simulink model "gates"  (R2024a)
settings: Solver=VariableStepAuto  StartTime=0.0  StopTime=10.0  RelTol=1e-3
libraries: simulink x6
settings Model: Creator=lokes  LastModifiedBy=tusha
settings RTWCC: GPUComputeCapability=3.5

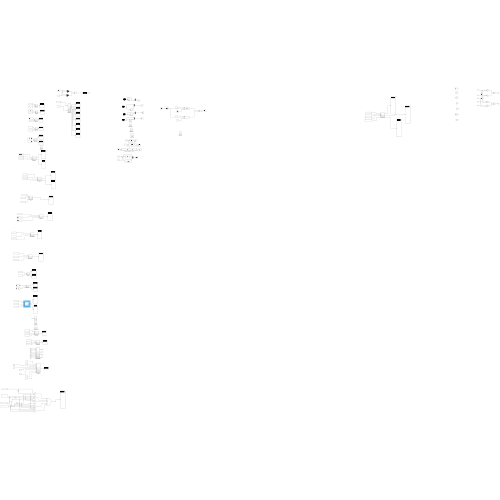
[thumbnail: Simulink's stored preview of the top-level diagram]
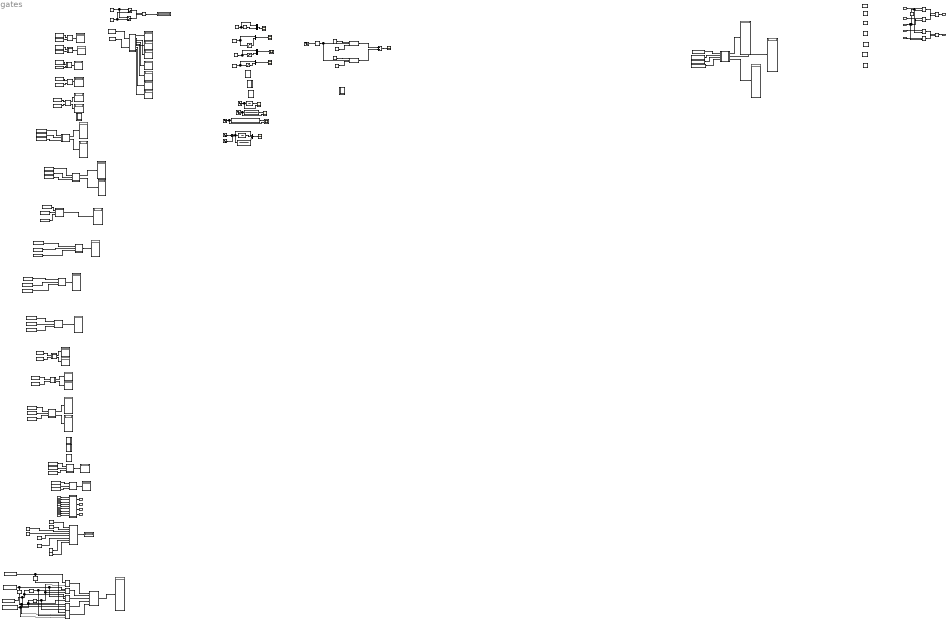
== system gates ==
  note: [numd, dend]=bilinear([1],[1 1.414 1],1)
  In1 : Inport
  In2 : Inport  Port=2
  In3 : Inport  Port=3
  In4 : Inport  Port=4
  In5 : Inport  Port=5
  In6 : Inport  Port=6
  In7 : Inport  Port=7
  In8 : Inport  Port=8
  In10 : Inport  Port=9
  In9 : Inport  Port=10
  In11 : Inport  Port=11
  In12 : Inport  Port=12
  In13 : Inport  Port=13
  In14 : Inport  Port=14
  2:1MUX(Basic) : Subsystem
  2:1MUX(NAND) : Subsystem
  3NOR USING 2NOR : Subsystem
  4:1MUX : Subsystem
  4BIT(2:1)MUXNAND : Subsystem
  A+B+C : Subsystem
  ABC : Subsystem
  AC+B : Subsystem
  Absorption : Subsystem
  Add : Sum
  BASIC GATES : Subsystem
  Bus Creator{,1..3} (4 alike) : BusCreator  Inputs=2
  Bus Creator4 : BusCreator  Inputs=3
  Constant{,40..41,55} (4 alike) : Constant  Value=0
  Constant{1,39,49..54,56} (9 alike) : Constant
  Constant{2,4,6,8,10,12,32,34,45,48} (10 alike) : Constant  Value=[0 0 1 1]
  Constant{3,5,7,9,11,13,33,35} (8 alike) : Constant  Value=[0 1 0 1]
  Constant{14,17,20,23,26,29,36} (7 alike) : Constant  Value=[0 0 0 0 1 1 1 1]
  Constant{15,18,21,24,27,30,37} (7 alike) : Constant  Value=[0 0 1 1 0 0 1 1]
  Constant{16,19,22,25,28,31,38} (7 alike) : Constant  Value=[0 1 0 1 0 1 0 1]
  Constant42 : Constant  Value=-1
  Constant43 : Constant  Value=[0 1 0 0]
  Constant44 : Constant  Value=[0 0 0 1]
  Constant46 : Constant  Value=[0 1 0 0]
  Constant47 : Constant  Value=[0 0 0 1]
  Constant57 : Constant  Value=[0 0 0 0 0 0 0 0 1 1 1 1 1 1 1 1]
  Constant58 : Constant  Value=[0 0 0 0 1 1 1 1 0 0 0 0 1 1 1 1]
  Constant59 : Constant  Value=[0 0 1 1 0 0 1 1 0 0 1 1 0 0 1 1]
  Constant60 : Constant  Value=[0 1 0 1 0 1 0 1 0 1 0 1 0 1 0 1]
  Constant61 : Constant  Value=[0 0 0 0 0 0 0 0 1 1 1 1 1 1 1 1]
  Constant62 : Constant  Value=[0 0 0 0 1 1 1 1 0 0 0 0 1 1 1 1]
  Constant63 : Constant  Value=[0 0 1 1 0 0 1 1 0 0 1 1 0 0 1 1]
  Constant64 : Constant  Value=[0 1 0 1 0 1 0 1 0 1 0 1 0 1 0 1]
  DeMorgan : Subsystem
  Deadzone : DeadZone  LowerValue=-0.25  UpperValue=0.25
  Discrete Transfer Fcn : DiscreteTransferFcn  Numerator=[1 1]  Denominator=[3 -1]
  Discrete Transfer Fcn1 : DiscreteTransferFcn  Numerator=[7.828 -6 2.171]  Denominator=[1 2 1]
  Discrete Zero-Pole : DiscreteZeroPole  Zeros=[-1 -1]  Poles=[0.383-0.36i 0.383+0.36i]  Gain=1/7.828  SampleTime=-1
  Display{,1..34} (35 alike) : Display
  Distributive : Subsystem
  Double Clip : Saturate
  FULLADDER_BASIC : Subsystem
  Fullwave rectifier : Subsystem
  HA_Basic : Subsystem
  HalfAdder_PulseIP : Subsystem
  Halfadder_NAND : Subsystem
  HalfwaveRectifier : Subsystem
  Inrementer : Subsystem
  Logical Operator : Logic  Operator=XOR  AllPortsSameDT=off  OutDataTypeStr=boolean
  Logical Operator1 : Logic  Operator=XOR  IconShape=distinctive  AllPortsSameDT=off  OutDataTypeStr=boolean
  Logical Operator10 : Logic  Operator=OR  IconShape=distinctive  AllPortsSameDT=off  OutDataTypeStr=boolean
  Logical Operator11 : Logic  Operator=OR  IconShape=distinctive  AllPortsSameDT=off  OutDataTypeStr=boolean
  Logical Operator{2,8..9,12..13,15} (6 alike) : Logic  IconShape=distinctive  AllPortsSameDT=off  OutDataTypeStr=boolean
  Logical Operator{7,14,21..24} (6 alike) : Logic  Operator=NOT  IconShape=distinctive  AllPortsSameDT=off  OutDataTypeStr=boolean
  Logical Operator16 : Logic  Inputs=3  IconShape=distinctive  AllPortsSameDT=off  OutDataTypeStr=boolean
  Logical Operator17 : Logic  Inputs=3  IconShape=distinctive  AllPortsSameDT=off  OutDataTypeStr=boolean
  Logical Operator18 : Logic  Inputs=3  IconShape=distinctive  AllPortsSameDT=off  OutDataTypeStr=boolean
  Logical Operator19 : Logic  Inputs=4  IconShape=distinctive  AllPortsSameDT=off  OutDataTypeStr=boolean
  Logical Operator20 : Logic  Operator=OR  Inputs=5  IconShape=distinctive  AllPortsSameDT=off  OutDataTypeStr=boolean
  Logical Operator3 : Logic  Operator=NAND  IconShape=distinctive  AllPortsSameDT=off  OutDataTypeStr=boolean
  Logical Operator4 : Logic  Operator=OR  IconShape=distinctive  AllPortsSameDT=off  OutDataTypeStr=boolean
  Logical Operator5 : Logic  Operator=NOR  IconShape=distinctive  AllPortsSameDT=off  OutDataTypeStr=boolean
  Logical Operator6 : Logic  Operator=NXOR  IconShape=distinctive  AllPortsSameDT=off  OutDataTypeStr=boolean
  Manual Switch : ManualSwitch  CurrentSetting=0
  Manual Switch1 : ManualSwitch  CurrentSetting=0
  Negative Clip : Saturate  UpperLimit=1
  Positive Clip : Saturate  LowerLimit=-1
  PulseIP_XOR : Subsystem
  Rate Limitter : Subsystem
  Saturation Dynamic : simulink/Discontinuities/Saturation Dynamic  OutMin=[]  OutMax=[]  OutDataTypeStr=Inherit: Same as second input  OutDataType=fixdt(1, 16)  OutScaling=2^-10  DoSatur=off
  Saturation Dynamic1 : simulink/Discontinuities/Saturation Dynamic  OutMin=[]  OutMax=[]  OutDataTypeStr=Inherit: Same as second input  OutDataType=fixdt(1, 16)  OutScaling=2^-10  DoSatur=off
  Scope{,1..4,8} (6 alike) : Scope
  Scope5 : Scope  NumInputPorts=2
  Scope6 : Scope  NumInputPorts=2
  Scope7 : Scope  NumInputPorts=2
  Signal Generator : SignalGenerator  Units=rad/sec
  Signal Generator2 : SignalGenerator  Units=rad/sec
  Signal Generator3 : SignalGenerator  Units=rad/sec
  Signal Generator4 : SignalGenerator  Frequency=0.2  Units=rad/sec
  Sine Wave{,1..4} (5 alike) : Sin  SampleTime=0
  Sine Wave5 : Sin  Frequency=10  SampleTime=0
  Sum : Sum  Inputs=|++
  Transfer Fcn : TransferFcn  Numerator=[2]  Denominator=[1 2]
  Transfer Fcn1 : TransferFcn  Denominator=[1 1.414 1]
  Transport Delay1 : TransportDelay  DelayTime=3
  Transport Delay : Subsystem
  X(Y+Z)+XY : Subsystem
  XNOR_NOR : Subsystem
  XOR_NOR : Subsystem
  XOR_Nand : Subsystem
  XOR_basic : Subsystem
  XYZ : Subsystem
  Out1 : Outport
  Out2 : Outport  Port=2
  Out3 : Outport  Port=3
  Out4 : Outport  Port=4
  Out5 : Outport  Port=5
  Out6 : Outport  Port=6
  wires:
  Logical Operator/1 -> Display/1
  Constant/1 -> Manual Switch1/1, Manual Switch/1
  Constant1/1 -> Manual Switch/2, Manual Switch1/2
  Manual Switch/1 -> Logical Operator/1
  Manual Switch1/1 -> Logical Operator/2
  Constant2/1 -> BASIC GATES/1(In1)
  Constant3/1 -> BASIC GATES/2(In2)
  BASIC GATES/1(Out1) -> Display1/1
  BASIC GATES/2(Out2) -> Display2/1
  BASIC GATES/3(Out3) -> Display3/1
  BASIC GATES/4(Out4) -> Display4/1
  BASIC GATES/5(Out5) -> Display5/1
  BASIC GATES/6(Out6) -> Display6/1
  BASIC GATES/7(Out7) -> Display7/1
  Constant4/1 -> XOR_basic/1(In1)
  Constant5/1 -> XOR_basic/2(In2)
  XOR_basic/1(Out1) -> Display8/1
  Constant6/1 -> XOR_Nand/1(In1)
  Constant7/1 -> XOR_Nand/2(In2)
  XOR_Nand/1(Out1) -> Display9/1
  Constant8/1 -> XNOR_NOR/1(In1)
  Constant9/1 -> XNOR_NOR/2(In2)
  XNOR_NOR/1(Out1) -> Display10/1
  Constant10/1 -> XOR_NOR/1(In1)
  Constant11/1 -> XOR_NOR/2(In2)
  XOR_NOR/1(Out1) -> Display11/1
  Constant12/1 -> DeMorgan/1(In1)
  Constant13/1 -> DeMorgan/2(In2)
  DeMorgan/1(Out1) -> Display12/1
  DeMorgan/2(Out2) -> Display13/1
  Constant14/1 -> Distributive/1(In1)
  Constant15/1 -> Distributive/2(In2)
  Constant16/1 -> Distributive/3(In3)
  Distributive/1(Out1) -> Display15/1
  Distributive/2(Out2) -> Display14/1
  Constant17/1 -> AC+B/1(In1)
  Constant18/1 -> AC+B/2(In2)
  Constant19/1 -> AC+B/3(In3)
  AC+B/1(Out1) -> Display17/1
  AC+B/2(Out2) -> Display16/1
  Constant20/1 -> ABC/1(In1)
  Constant21/1 -> ABC/2(In2)
  Constant22/1 -> ABC/3(In3)
  ABC/1(Out1) -> Display18/1
  Constant23/1 -> A+B+C/1(In1)
  Constant24/1 -> A+B+C/2(In2)
  Constant25/1 -> A+B+C/3(In3)
  A+B+C/1(Out1) -> Display19/1
  Constant26/1 -> 3NOR USING 2NOR/1(In1)
  Constant27/1 -> 3NOR USING 2NOR/2(In2)
  Constant28/1 -> 3NOR USING 2NOR/3(In3)
  3NOR USING 2NOR/1(Out1) -> Display20/1
  Constant29/1 -> X(Y+Z)+XY/1(In1)
  Constant30/1 -> X(Y+Z)+XY/2(In2)
  Constant31/1 -> X(Y+Z)+XY/3(In3)
  X(Y+Z)+XY/1(Out1) -> Display21/1
  Constant32/1 -> HA_Basic/1(In1)
  Constant33/1 -> HA_Basic/2(In2)
  HA_Basic/1(Out1) -> Display22/1
  HA_Basic/2(Out2) -> Display23/1
  Constant34/1 -> Halfadder_NAND/1(In1)
  Constant35/1 -> Halfadder_NAND/2(In2)
  Halfadder_NAND/1(Out1) -> Display24/1
  Halfadder_NAND/2(Out2) -> Display25/1
  Constant36/1 -> FULLADDER_BASIC/1(In1)
  Constant37/1 -> FULLADDER_BASIC/2(In2)
  Constant38/1 -> FULLADDER_BASIC/3(In3)
  FULLADDER_BASIC/1(Out1) -> Display27/1
  FULLADDER_BASIC/2(Out2) -> Display26/1
  Deadzone/1 -> Bus Creator3/2
  Negative Clip/1 -> Bus Creator2/2
  Signal Generator4/1 -> Bus Creator3/1, Deadzone/1
  Double Clip/1 -> Bus Creator/2
  Signal Generator2/1 -> Bus Creator1/1, Positive Clip/1
  Signal Generator/1 -> Bus Creator/1, Double Clip/1
  Bus Creator/1 -> Scope/1
  Signal Generator3/1 -> Bus Creator2/1, Negative Clip/1
  Bus Creator1/1 -> Scope2/1
  Positive Clip/1 -> Bus Creator1/2
  Bus Creator2/1 -> Scope3/1
  Bus Creator3/1 -> Scope4/1
  Sine Wave/1 -> Transport Delay1/1
  Constant39/1 -> Saturation Dynamic/1
  Constant40/1 -> Saturation Dynamic/3
  Saturation Dynamic/1 -> Add/1
  Saturation Dynamic1/1 -> Add/2
  Constant41/1 -> Saturation Dynamic1/1
  Constant42/1 -> Saturation Dynamic1/3
  Transport Delay1/1 -> Saturation Dynamic1/2, Saturation Dynamic/2
  Add/1 -> Scope1/1
  Constant43/1 -> 2:1MUX(Basic)/1(In1)
  Constant44/1 -> 2:1MUX(Basic)/2(In2)
  Constant45/1 -> 2:1MUX(Basic)/3(In3)
  2:1MUX(Basic)/1(Out1) -> Display28/1
  Constant46/1 -> 2:1MUX(NAND)/1(In1)
  Constant47/1 -> 2:1MUX(NAND)/2(In2)
  Constant48/1 -> 2:1MUX(NAND)/3(In3)
  2:1MUX(NAND)/1(Out1) -> Display29/1
  In1/1 -> Logical Operator8/1
  In2/1 -> Logical Operator9/1
  In3/1 -> Logical Operator12/1
  In4/1 -> Logical Operator13/1
  In5/1 -> Logical Operator13/2, Logical Operator9/2, Logical Operator14/1
  Logical Operator14/1 -> Logical Operator12/2, Logical Operator8/2
  Logical Operator8/1 -> Logical Operator10/1
  Logical Operator9/1 -> Logical Operator10/2
  Logical Operator12/1 -> Logical Operator11/1
  Logical Operator13/1 -> Logical Operator11/2
  Logical Operator10/1 -> Out1/1
  Logical Operator11/1 -> Out2/1
  In10/1 -> 4BIT(2:1)MUXNAND/4(In10)
  In9/1 -> 4BIT(2:1)MUXNAND/5(In4)
  In8/1 -> 4BIT(2:1)MUXNAND/3(In7)
  In11/1 -> 4BIT(2:1)MUXNAND/6(In3)
  In6/1 -> 4BIT(2:1)MUXNAND/1(In2)
  4BIT(2:1)MUXNAND/1(Out1) -> Out3/1
  In13/1 -> 4BIT(2:1)MUXNAND/8(In12)
  4BIT(2:1)MUXNAND/4(Out2) -> Out6/1
  In14/1 -> 4BIT(2:1)MUXNAND/9(In6)
  4BIT(2:1)MUXNAND/2(Out3) -> Out4/1
  In12/1 -> 4BIT(2:1)MUXNAND/7(In9)
  4BIT(2:1)MUXNAND/3(Out4) -> Out5/1
  In7/1 -> 4BIT(2:1)MUXNAND/2(In1)
  Constant49/1 -> 4:1MUX/1(In15)
  Constant50/1 -> 4:1MUX/2(In16)
  Constant51/1 -> 4:1MUX/3(In17)
  Constant53/1 -> 4:1MUX/5(In19)
  Constant54/1 -> 4:1MUX/6(In20)
  Constant55/1 -> 4:1MUX/7(In21)
  Constant56/1 -> 4:1MUX/8(In22)
  4:1MUX/1(Out7) -> Display30/1
  Constant52/1 -> 4:1MUX/4(In18)
  Logical Operator15/1 -> Logical Operator20/1
  Logical Operator17/1 -> Logical Operator20/3
  Logical Operator19/1 -> Logical Operator20/5
  Logical Operator21/1 -> Logical Operator18/3, Logical Operator15/2, Logical Operator16/3
  Logical Operator16/1 -> Logical Operator20/2
  Constant57/1 -> Logical Operator24/1, Logical Operator15/1
  Constant58/1 -> Logical Operator23/1, Logical Operator17/1, Logical Operator16/1
  Logical Operator18/1 -> Logical Operator20/4
  Constant60/1 -> Logical Operator19/4, Logical Operator21/1, Logical Operator17/3
  Constant59/1 -> Logical Operator18/2, Logical Operator22/1, Logical Operator17/2
  Logical Operator22/1 -> Logical Operator19/3, Logical Operator16/2
  Logical Operator23/1 -> Logical Operator19/2, Logical Operator18/1
  Logical Operator24/1 -> Logical Operator19/1
  Logical Operator20/1 -> Display31/1
  Discrete Transfer Fcn/1 -> Scope5/1
  Sine Wave1/1 -> Scope5/2, Discrete Transfer Fcn/1
  Sine Wave2/1 -> Scope6/2, Discrete Transfer Fcn1/1
  Discrete Transfer Fcn1/1 -> Scope6/1
  Discrete Zero-Pole/1 -> Scope7/1
  Sine Wave3/1 -> Discrete Zero-Pole/1, Scope7/2
  Sine Wave4/1 -> Sum/1
  Sine Wave5/1 -> Sum/2
  Sum/1 -> Transfer Fcn1/1, Bus Creator4/1, Transfer Fcn/1
  Bus Creator4/1 -> Scope8/1
  Transfer Fcn/1 -> Bus Creator4/2
  Transfer Fcn1/1 -> Bus Creator4/3
  Constant61/1 -> XYZ/1(In1)
  Constant62/1 -> XYZ/2(In2)
  Constant63/1 -> XYZ/3(In3)
  Constant64/1 -> XYZ/4(In4)
  XYZ/1(Out1) -> Display32/1
  XYZ/2(Out2) -> Display33/1
  XYZ/3(Out3) -> Display34/1

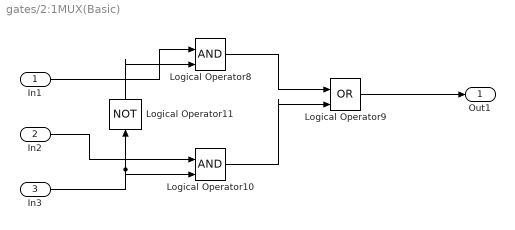
== system gates/2:1MUX(Basic) ==
  In1 : Inport
  In2 : Inport  Port=2
  In3 : Inport  Port=3
  Logical Operator10 : Logic  IconShape=distinctive  AllPortsSameDT=off  OutDataTypeStr=boolean
  Logical Operator11 : Logic  Operator=NOT  IconShape=distinctive  AllPortsSameDT=off  OutDataTypeStr=boolean
  Logical Operator8 : Logic  IconShape=distinctive  AllPortsSameDT=off  OutDataTypeStr=boolean
  Logical Operator9 : Logic  Operator=OR  IconShape=distinctive  AllPortsSameDT=off  OutDataTypeStr=boolean
  Out1 : Outport
  wires:
  In2/1 -> Logical Operator10/1
  Logical Operator8/1 -> Logical Operator9/1
  Logical Operator9/1 -> Out1/1
  In1/1 -> Logical Operator8/1
  Logical Operator10/1 -> Logical Operator9/2
  Logical Operator11/1 -> Logical Operator8/2
  In3/1 -> Logical Operator10/2, Logical Operator11/1

== system gates/2:1MUX(NAND) ==
  In1 : Inport
  In2 : Inport  Port=2
  In3 : Inport  Port=3
  Logical Operator{8..11} (4 alike) : Logic  Operator=NAND  IconShape=distinctive  AllPortsSameDT=off  OutDataTypeStr=boolean
  Out1 : Outport
  wires:
  Logical Operator10/1 -> Logical Operator11/2
  In3/1 -> Logical Operator8/2, Logical Operator8/1, Logical Operator10/2
  In2/1 -> Logical Operator10/1
  Logical Operator8/1 -> Logical Operator9/1
  In1/1 -> Logical Operator9/2
  Logical Operator9/1 -> Logical Operator11/1
  Logical Operator11/1 -> Out1/1

== system gates/3NOR USING 2NOR ==
  In1 : Inport
  In2 : Inport  Port=2
  In3 : Inport  Port=3
  Logical Operator1 : Logic  Operator=NOR  IconShape=distinctive  AllPortsSameDT=off  OutDataTypeStr=boolean
  Logical Operator2 : Logic  Operator=NOR  IconShape=distinctive  AllPortsSameDT=off  OutDataTypeStr=boolean
  Logical Operator5 : Logic  Operator=NOR  IconShape=distinctive  AllPortsSameDT=off  OutDataTypeStr=boolean
  Out1 : Outport
  wires:
  Logical Operator1/1 -> Logical Operator2/1
  Logical Operator5/1 -> Logical Operator1/2, Logical Operator1/1
  In2/1 -> Logical Operator5/2
  Logical Operator2/1 -> Out1/1
  In1/1 -> Logical Operator5/1
  In3/1 -> Logical Operator2/2

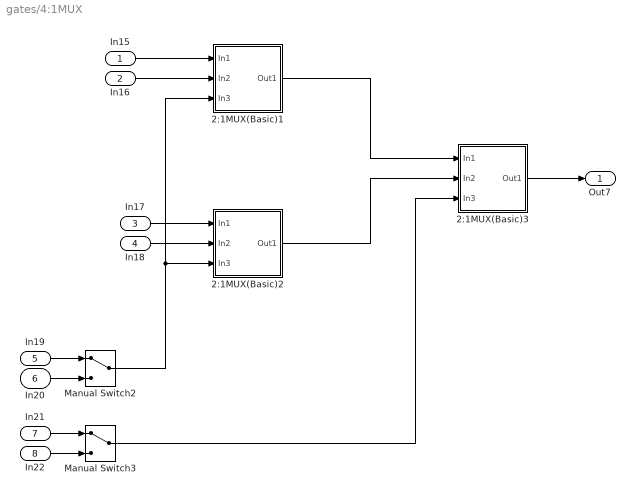
== system gates/4:1MUX ==
  In15 : Inport
  In16 : Inport  Port=2
  In17 : Inport  Port=3
  In18 : Inport  Port=4
  In19 : Inport  Port=5
  In20 : Inport  Port=6
  In21 : Inport  Port=7
  In22 : Inport  Port=8
  2:1MUX(Basic)1 : Subsystem
  2:1MUX(Basic)2 : Subsystem
  2:1MUX(Basic)3 : Subsystem
  Manual Switch2 : ManualSwitch
  Manual Switch3 : ManualSwitch
  Out7 : Outport
  wires:
  In18/1 -> 2:1MUX(Basic)2/2(In2)
  In16/1 -> 2:1MUX(Basic)1/2(In2)
  In17/1 -> 2:1MUX(Basic)2/1(In1)
  Manual Switch2/1 -> 2:1MUX(Basic)1/3(In3), 2:1MUX(Basic)2/3(In3)
  2:1MUX(Basic)2/1(Out1) -> 2:1MUX(Basic)3/2(In2)
  2:1MUX(Basic)1/1(Out1) -> 2:1MUX(Basic)3/1(In1)
  In19/1 -> Manual Switch2/1
  In20/1 -> Manual Switch2/2
  Manual Switch3/1 -> 2:1MUX(Basic)3/3(In3)
  In15/1 -> 2:1MUX(Basic)1/1(In1)
  In22/1 -> Manual Switch3/2
  In21/1 -> Manual Switch3/1
  2:1MUX(Basic)3/1(Out1) -> Out7/1

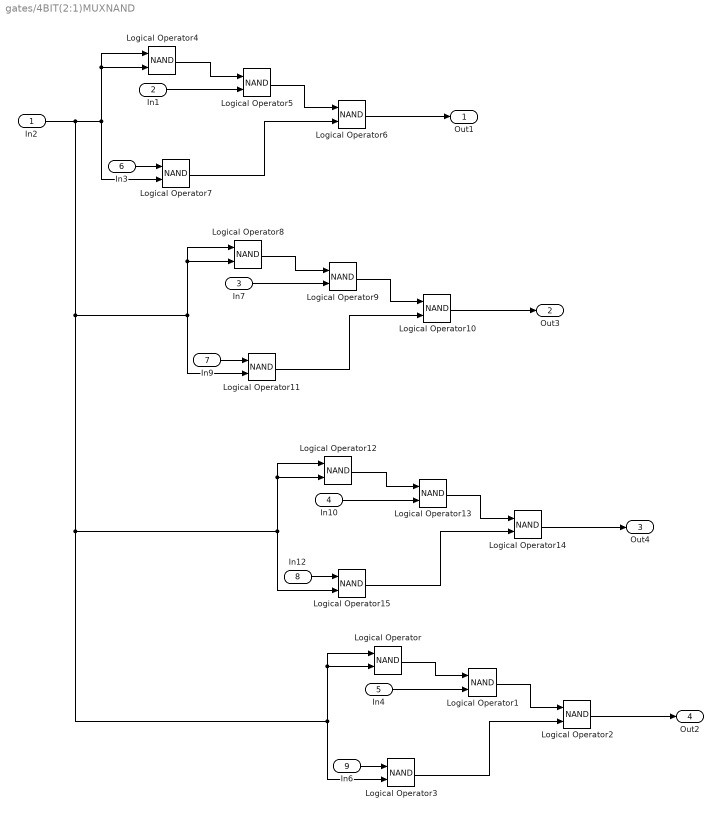
== system gates/4BIT(2:1)MUXNAND ==
  In2 : Inport
  In1 : Inport  Port=2
  In7 : Inport  Port=3
  In10 : Inport  Port=4
  In4 : Inport  Port=5
  In3 : Inport  Port=6
  In9 : Inport  Port=7
  In12 : Inport  Port=8
  In6 : Inport  Port=9
  Logical Operator{,1..15} (16 alike) : Logic  Operator=NAND  AllPortsSameDT=off  OutDataTypeStr=boolean
  Out1 : Outport
  Out3 : Outport  Port=2
  Out4 : Outport  Port=3
  Out2 : Outport  Port=4
  wires:
  In12/1 -> Logical Operator15/1
  Logical Operator/1 -> Logical Operator1/1
  In2/1 -> Logical Operator/2, Logical Operator/1, Logical Operator3/2, Logical Operator12/2, Logical Operator12/1, Logical Operator15/2, Logical Operator8/2, Logical Operator8/1, Logical Operator11/2, Logical Operator4/2, Logical Operator4/1, Logical Operator7/2
  Logical Operator14/1 -> Out4/1
  In10/1 -> Logical Operator13/2
  Logical Operator7/1 -> Logical Operator6/2
  Logical Operator5/1 -> Logical Operator6/1
  Logical Operator2/1 -> Out2/1
  Logical Operator13/1 -> Logical Operator14/1
  Logical Operator15/1 -> Logical Operator14/2
  Logical Operator12/1 -> Logical Operator13/1
  In9/1 -> Logical Operator11/1
  In7/1 -> Logical Operator9/2
  Logical Operator11/1 -> Logical Operator10/2
  Logical Operator9/1 -> Logical Operator10/1
  Logical Operator8/1 -> Logical Operator9/1
  Logical Operator10/1 -> Out3/1
  Logical Operator4/1 -> Logical Operator5/1
  In6/1 -> Logical Operator3/1
  Logical Operator3/1 -> Logical Operator2/2
  Logical Operator6/1 -> Out1/1
  Logical Operator1/1 -> Logical Operator2/1
  In4/1 -> Logical Operator1/2
  In1/1 -> Logical Operator5/2
  In3/1 -> Logical Operator7/1

== system gates/A+B+C ==
  In1 : Inport
  In2 : Inport  Port=2
  In3 : Inport  Port=3
  Logical Operator{3,6..8} (4 alike) : Logic  Operator=NOR  IconShape=distinctive  AllPortsSameDT=off  OutDataTypeStr=boolean
  Out1 : Outport
  wires:
  Logical Operator3/1 -> Logical Operator6/2, Logical Operator6/1
  In2/1 -> Logical Operator3/2
  Logical Operator7/1 -> Logical Operator8/2, Logical Operator8/1
  In1/1 -> Logical Operator3/1
  Logical Operator6/1 -> Logical Operator7/1
  Logical Operator8/1 -> Out1/1
  In3/1 -> Logical Operator7/2

== system gates/ABC ==
  In1 : Inport
  In2 : Inport  Port=2
  In3 : Inport  Port=3
  Logical Operator{1..4} (4 alike) : Logic  Operator=NAND  IconShape=distinctive  AllPortsSameDT=off  OutDataTypeStr=boolean
  Out1 : Outport
  wires:
  Logical Operator4/1 -> Out1/1
  Logical Operator2/1 -> Logical Operator4/2, Logical Operator4/1
  Logical Operator3/1 -> Logical Operator1/2, Logical Operator1/1
  In3/1 -> Logical Operator2/2
  Logical Operator1/1 -> Logical Operator2/1
  In1/1 -> Logical Operator3/1
  In2/1 -> Logical Operator3/2

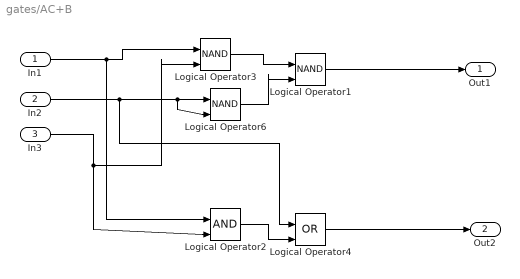
== system gates/AC+B ==
  In1 : Inport
  In2 : Inport  Port=2
  In3 : Inport  Port=3
  Logical Operator1 : Logic  Operator=NAND  IconShape=distinctive  AllPortsSameDT=off  OutDataTypeStr=boolean
  Logical Operator2 : Logic  IconShape=distinctive  AllPortsSameDT=off  OutDataTypeStr=boolean
  Logical Operator3 : Logic  Operator=NAND  IconShape=distinctive  AllPortsSameDT=off  OutDataTypeStr=boolean
  Logical Operator4 : Logic  Operator=OR  IconShape=distinctive  AllPortsSameDT=off  OutDataTypeStr=boolean
  Logical Operator6 : Logic  Operator=NAND  IconShape=distinctive  AllPortsSameDT=off  OutDataTypeStr=boolean
  Out1 : Outport
  Out2 : Outport  Port=2
  wires:
  Logical Operator6/1 -> Logical Operator1/2
  Logical Operator1/1 -> Out1/1
  In2/1 -> Logical Operator6/2, Logical Operator6/1, Logical Operator4/1
  In1/1 -> Logical Operator3/1, Logical Operator2/1
  In3/1 -> Logical Operator3/2, Logical Operator2/2
  Logical Operator2/1 -> Logical Operator4/2
  Logical Operator4/1 -> Out2/1
  Logical Operator3/1 -> Logical Operator1/1

== system gates/Absorption ==
  Constant14 : Constant  Value=[0 0 1 1]
  Constant15 : Constant  Value=[0 1 0 1]
  Display14 : Display
  Display15 : Display
  Logical Operator2 : Logic  IconShape=distinctive  AllPortsSameDT=off  OutDataTypeStr=boolean
  Logical Operator4 : Logic  Operator=OR  IconShape=distinctive  AllPortsSameDT=off  OutDataTypeStr=boolean
  wires:
  Constant15/1 -> Logical Operator4/2
  Logical Operator2/1 -> Display15/1
  Constant14/1 -> Logical Operator2/1, Logical Operator4/1, Display14/1
  Logical Operator4/1 -> Logical Operator2/2

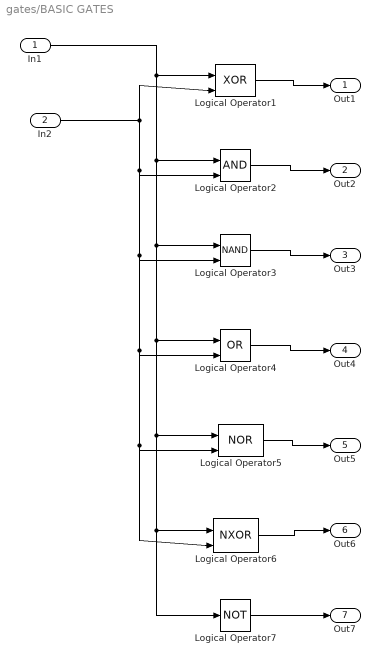
== system gates/BASIC GATES ==
  In1 : Inport
  In2 : Inport  Port=2
  Logical Operator1 : Logic  Operator=XOR  IconShape=distinctive  AllPortsSameDT=off  OutDataTypeStr=boolean
  Logical Operator2 : Logic  IconShape=distinctive  AllPortsSameDT=off  OutDataTypeStr=boolean
  Logical Operator3 : Logic  Operator=NAND  IconShape=distinctive  AllPortsSameDT=off  OutDataTypeStr=boolean
  Logical Operator4 : Logic  Operator=OR  IconShape=distinctive  AllPortsSameDT=off  OutDataTypeStr=boolean
  Logical Operator5 : Logic  Operator=NOR  IconShape=distinctive  AllPortsSameDT=off  OutDataTypeStr=boolean
  Logical Operator6 : Logic  Operator=NXOR  IconShape=distinctive  AllPortsSameDT=off  OutDataTypeStr=boolean
  Logical Operator7 : Logic  Operator=NOT  IconShape=distinctive  AllPortsSameDT=off  OutDataTypeStr=boolean
  Out1 : Outport
  Out2 : Outport  Port=2
  Out3 : Outport  Port=3
  Out4 : Outport  Port=4
  Out5 : Outport  Port=5
  Out6 : Outport  Port=6
  Out7 : Outport  Port=7
  wires:
  In2/1 -> Logical Operator6/2, Logical Operator5/2, Logical Operator4/2, Logical Operator3/2, Logical Operator2/2, Logical Operator1/2
  Logical Operator7/1 -> Out7/1
  Logical Operator1/1 -> Out1/1
  In1/1 -> Logical Operator3/1, Logical Operator4/1, Logical Operator7/1, Logical Operator6/1, Logical Operator5/1, Logical Operator2/1, Logical Operator1/1
  Logical Operator4/1 -> Out4/1
  Logical Operator6/1 -> Out6/1
  Logical Operator5/1 -> Out5/1
  Logical Operator2/1 -> Out2/1
  Logical Operator3/1 -> Out3/1

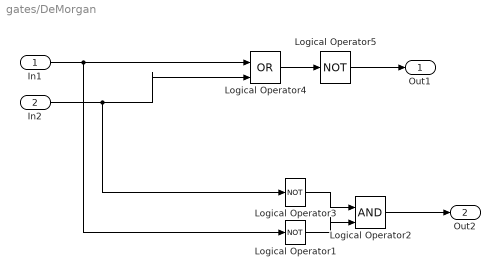
== system gates/DeMorgan ==
  In1 : Inport
  In2 : Inport  Port=2
  Logical Operator1 : Logic  Operator=NOT  IconShape=distinctive  AllPortsSameDT=off  OutDataTypeStr=boolean
  Logical Operator2 : Logic  IconShape=distinctive  AllPortsSameDT=off  OutDataTypeStr=boolean
  Logical Operator3 : Logic  Operator=NOT  IconShape=distinctive  AllPortsSameDT=off  OutDataTypeStr=boolean
  Logical Operator4 : Logic  Operator=OR  IconShape=distinctive  AllPortsSameDT=off  OutDataTypeStr=boolean
  Logical Operator5 : Logic  Operator=NOT  IconShape=distinctive  AllPortsSameDT=off  OutDataTypeStr=boolean
  Out1 : Outport
  Out2 : Outport  Port=2
  wires:
  In2/1 -> Logical Operator3/1, Logical Operator4/2
  Logical Operator5/1 -> Out1/1
  Logical Operator1/1 -> Logical Operator2/2
  Logical Operator2/1 -> Out2/1
  Logical Operator3/1 -> Logical Operator2/1
  In1/1 -> Logical Operator1/1, Logical Operator4/1
  Logical Operator4/1 -> Logical Operator5/1

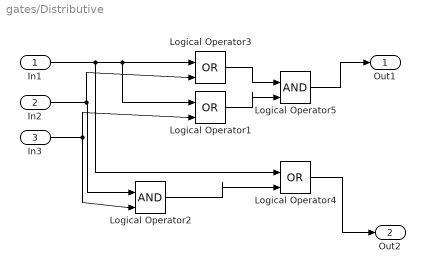
== system gates/Distributive ==
  In1 : Inport
  In2 : Inport  Port=2
  In3 : Inport  Port=3
  Logical Operator1 : Logic  Operator=OR  IconShape=distinctive  AllPortsSameDT=off  OutDataTypeStr=boolean
  Logical Operator2 : Logic  IconShape=distinctive  AllPortsSameDT=off  OutDataTypeStr=boolean
  Logical Operator3 : Logic  Operator=OR  IconShape=distinctive  AllPortsSameDT=off  OutDataTypeStr=boolean
  Logical Operator4 : Logic  Operator=OR  IconShape=distinctive  AllPortsSameDT=off  OutDataTypeStr=boolean
  Logical Operator5 : Logic  IconShape=distinctive  AllPortsSameDT=off  OutDataTypeStr=boolean
  Out1 : Outport
  Out2 : Outport  Port=2
  wires:
  In3/1 -> Logical Operator2/2, Logical Operator1/2
  Logical Operator5/1 -> Out1/1
  In2/1 -> Logical Operator3/2, Logical Operator2/1
  Logical Operator2/1 -> Logical Operator4/2
  Logical Operator3/1 -> Logical Operator5/1
  Logical Operator1/1 -> Logical Operator5/2
  In1/1 -> Logical Operator1/1, Logical Operator3/1, Logical Operator4/1
  Logical Operator4/1 -> Out2/1

== system gates/FULLADDER_BASIC ==
  In1 : Inport
  In2 : Inport  Port=2
  In3 : Inport  Port=3
  HA_Basic1 : Subsystem
  HA_Basic2 : Subsystem
  Logical Operator4 : Logic  Operator=OR  IconShape=distinctive  AllPortsSameDT=off  OutDataTypeStr=boolean
  Out1 : Outport
  Out2 : Outport  Port=2
  wires:
  HA_Basic1/1(Out1) -> HA_Basic2/1(In1)
  HA_Basic1/2(Out2) -> Logical Operator4/2
  HA_Basic2/2(Out2) -> Logical Operator4/1
  In1/1 -> HA_Basic1/1(In1)
  Logical Operator4/1 -> Out2/1
  In2/1 -> HA_Basic1/2(In2)
  HA_Basic2/1(Out1) -> Out1/1
  In3/1 -> HA_Basic2/2(In2)

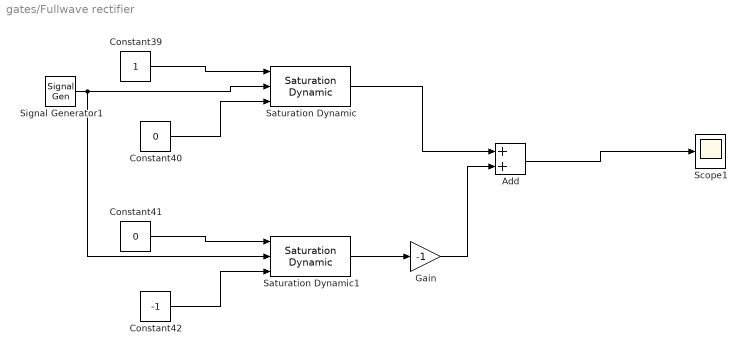
== system gates/Fullwave rectifier ==
  Add : Sum
  Constant39 : Constant
  Constant40 : Constant  Value=0
  Constant41 : Constant  Value=0
  Constant42 : Constant  Value=-1
  Gain : Gain  Gain=-1
  Saturation Dynamic : simulink/Discontinuities/Saturation Dynamic  OutMin=[]  OutMax=[]  OutDataTypeStr=Inherit: Same as second input  OutDataType=fixdt(1, 16)  OutScaling=2^-10  DoSatur=off
  Saturation Dynamic1 : simulink/Discontinuities/Saturation Dynamic  OutMin=[]  OutMax=[]  OutDataTypeStr=Inherit: Same as second input  OutDataType=fixdt(1, 16)  OutScaling=2^-10  DoSatur=off
  Scope1 : Scope
  Signal Generator1 : SignalGenerator  Units=rad/sec
  wires:
  Constant41/1 -> Saturation Dynamic1/1
  Gain/1 -> Add/2
  Constant39/1 -> Saturation Dynamic/1
  Constant42/1 -> Saturation Dynamic1/3
  Saturation Dynamic/1 -> Add/1
  Constant40/1 -> Saturation Dynamic/3
  Add/1 -> Scope1/1
  Saturation Dynamic1/1 -> Gain/1
  Signal Generator1/1 -> Saturation Dynamic1/2, Saturation Dynamic/2

== system gates/HA_Basic ==
  In1 : Inport
  In2 : Inport  Port=2
  Logical Operator2 : Logic  IconShape=distinctive  AllPortsSameDT=off  OutDataTypeStr=boolean
  XOR_basic1 : Subsystem
  Out1 : Outport
  Out2 : Outport  Port=2
  wires:
  XOR_basic1/1(Out1) -> Out1/1
  Logical Operator2/1 -> Out2/1
  In1/1 -> Logical Operator2/1, XOR_basic1/1(In1)
  In2/1 -> Logical Operator2/2, XOR_basic1/2(In2)

== system gates/HalfAdder_PulseIP ==
  Halfadder_NAND1 : Subsystem
  Pulse Generator : DiscretePulseGenerator  PulseType=Time based  PulseWidth=25
  Pulse Generator1 : DiscretePulseGenerator  PulseType=Time based  PulseWidth=50
  Scope5 : Scope  NumInputPorts=4
  wires:
  Halfadder_NAND1/2(Out2) -> Scope5/4
  Halfadder_NAND1/1(Out1) -> Scope5/3
  Pulse Generator1/1 -> Scope5/2, Halfadder_NAND1/2(In2)
  Pulse Generator/1 -> Scope5/1, Halfadder_NAND1/1(In1)

== system gates/Halfadder_NAND ==
  In1 : Inport
  In2 : Inport  Port=2
  Logical Operator1 : Logic  Operator=NAND  IconShape=distinctive  AllPortsSameDT=off  OutDataTypeStr=boolean
  Logical Operator3 : Logic  Operator=NAND  IconShape=distinctive  AllPortsSameDT=off  OutDataTypeStr=boolean
  XOR_Nand1 : Subsystem
  Out1 : Outport
  Out2 : Outport  Port=2
  wires:
  In2/1 -> Logical Operator3/2, XOR_Nand1/2(In2)
  Logical Operator3/1 -> Logical Operator1/2, Logical Operator1/1
  In1/1 -> Logical Operator3/1, XOR_Nand1/1(In1)
  XOR_Nand1/1(Out1) -> Out1/1
  Logical Operator1/1 -> Out2/1

== system gates/HalfwaveRectifier ==
  Constant39 : Constant
  Constant40 : Constant  Value=0
  Saturation Dynamic : simulink/Discontinuities/Saturation Dynamic  OutMin=[]  OutMax=[]  OutDataTypeStr=Inherit: Same as second input  OutDataType=fixdt(1, 16)  OutScaling=2^-10  DoSatur=off
  Scope1 : Scope  NumInputPorts=2
  Signal Generator1 : SignalGenerator  Units=rad/sec
  wires:
  Signal Generator1/1 -> Scope1/1, Saturation Dynamic/2
  Constant39/1 -> Saturation Dynamic/1
  Saturation Dynamic/1 -> Scope1/2
  Constant40/1 -> Saturation Dynamic/3

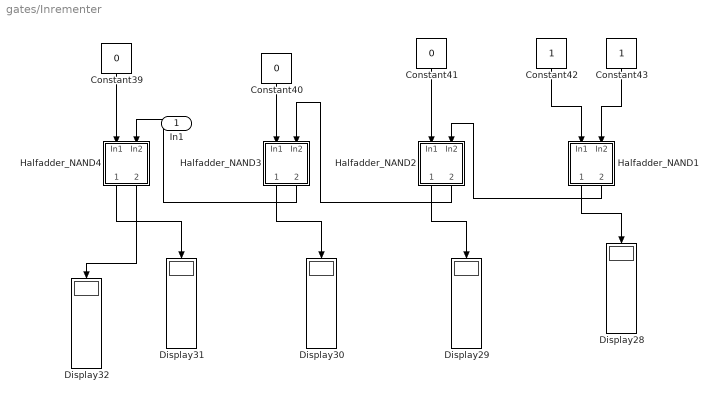
== system gates/Inrementer ==
  In1 : Inport
  Constant39 : Constant  Value=0
  Constant40 : Constant  Value=0
  Constant41 : Constant  Value=0
  Constant42 : Constant
  Constant43 : Constant
  Display{28..32} (5 alike) : Display
  Halfadder_NAND1 : Subsystem
  Halfadder_NAND2 : Subsystem
  Halfadder_NAND3 : Subsystem
  Halfadder_NAND4 : Subsystem
  wires:
  Halfadder_NAND2/1(Out1) -> Display29/1
  Constant39/1 -> Halfadder_NAND4/1(In1)
  Halfadder_NAND1/1(Out1) -> Display28/1
  Constant42/1 -> Halfadder_NAND1/1(In1)
  Halfadder_NAND2/2(Out2) -> Halfadder_NAND3/2(In2)
  Halfadder_NAND1/2(Out2) -> Halfadder_NAND2/2(In2)
  Constant43/1 -> Halfadder_NAND1/2(In2)
  Halfadder_NAND4/1(Out1) -> Display31/1
  Halfadder_NAND3/2(Out2) -> Halfadder_NAND4/2(In2)
  Halfadder_NAND3/1(Out1) -> Display30/1
  Constant40/1 -> Halfadder_NAND3/1(In1)
  Constant41/1 -> Halfadder_NAND2/1(In1)
  Halfadder_NAND4/2(Out2) -> Display32/1

== system gates/PulseIP_XOR ==
  Pulse Generator : DiscretePulseGenerator  PulseType=Time based  PulseWidth=50
  Pulse Generator1 : DiscretePulseGenerator  PulseType=Time based  PulseWidth=25
  Scope5 : Scope  NumInputPorts=3
  XOR_Nand1 : Subsystem
  wires:
  Pulse Generator1/1 -> Scope5/2, XOR_Nand1/2(In2)
  Pulse Generator/1 -> Scope5/1, XOR_Nand1/1(In1)
  XOR_Nand1/1(Out1) -> Scope5/3

== system gates/Rate Limitter ==
  Bus Creator4 : BusCreator  Inputs=2
  Constant43 : Constant
  Constant44 : Constant  Value=-1
  Rate Limiter Dynamic : simulink/Discontinuities/Rate Limiter Dynamic
  Scope5 : Scope
  Sine Wave1 : Sin  Amplitude=2  Frequency=2  SampleTime=0
  wires:
  Sine Wave1/1 -> Bus Creator4/2, Rate Limiter Dynamic/2
  Constant43/1 -> Rate Limiter Dynamic/1
  Constant44/1 -> Rate Limiter Dynamic/3
  Rate Limiter Dynamic/1 -> Bus Creator4/1
  Bus Creator4/1 -> Scope5/1

== system gates/Transport Delay ==
  Bus Creator4 : BusCreator  Inputs=2
  Scope1 : Scope
  Sine Wave : Sin  SampleTime=0
  Transport Delay : TransportDelay
  wires:
  Bus Creator4/1 -> Scope1/1
  Transport Delay/1 -> Bus Creator4/1
  Sine Wave/1 -> Bus Creator4/2, Transport Delay/1

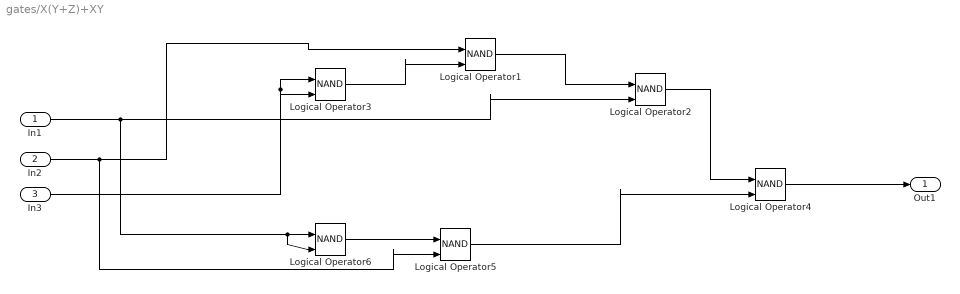
== system gates/X(Y+Z)+XY ==
  In1 : Inport
  In2 : Inport  Port=2
  In3 : Inport  Port=3
  Logical Operator{1..6} (6 alike) : Logic  Operator=NAND  IconShape=distinctive  AllPortsSameDT=off  OutDataTypeStr=boolean
  Out1 : Outport
  wires:
  In1/1 -> Logical Operator6/2, Logical Operator6/1, Logical Operator2/2
  In3/1 -> Logical Operator3/1, Logical Operator3/2
  In2/1 -> Logical Operator5/2, Logical Operator1/1
  Logical Operator5/1 -> Logical Operator4/2
  Logical Operator6/1 -> Logical Operator5/1
  Logical Operator3/1 -> Logical Operator1/2
  Logical Operator1/1 -> Logical Operator2/1
  Logical Operator2/1 -> Logical Operator4/1
  Logical Operator4/1 -> Out1/1

== system gates/XNOR_NOR ==
  In1 : Inport
  In2 : Inport  Port=2
  Logical Operator{1..3,5} (4 alike) : Logic  Operator=NOR  IconShape=distinctive  AllPortsSameDT=off  OutDataTypeStr=boolean
  Out1 : Outport
  wires:
  Logical Operator3/1 -> Out1/1
  Logical Operator2/1 -> Logical Operator3/2
  Logical Operator5/1 -> Logical Operator2/1, Logical Operator1/2
  In2/1 -> Logical Operator2/2, Logical Operator5/2
  In1/1 -> Logical Operator1/1, Logical Operator5/1
  Logical Operator1/1 -> Logical Operator3/1

== system gates/XOR_NOR ==
  In1 : Inport
  In2 : Inport  Port=2
  Logical Operator{1..5} (5 alike) : Logic  Operator=NOR  IconShape=distinctive  AllPortsSameDT=off  OutDataTypeStr=boolean
  Out1 : Outport
  wires:
  Logical Operator5/1 -> Logical Operator2/1, Logical Operator1/2
  In1/1 -> Logical Operator1/1, Logical Operator5/1
  In2/1 -> Logical Operator2/2, Logical Operator5/2
  Logical Operator3/1 -> Logical Operator4/1, Logical Operator4/2
  Logical Operator2/1 -> Logical Operator3/2
  Logical Operator1/1 -> Logical Operator3/1
  Logical Operator4/1 -> Out1/1

== system gates/XOR_Nand ==
  In1 : Inport
  In2 : Inport  Port=2
  Logical Operator{1..4} (4 alike) : Logic  Operator=NAND  IconShape=distinctive  AllPortsSameDT=off  OutDataTypeStr=boolean
  Out1 : Outport
  wires:
  Logical Operator4/1 -> Out1/1
  Logical Operator1/1 -> Logical Operator4/1
  Logical Operator3/1 -> Logical Operator2/1, Logical Operator1/2
  In2/1 -> Logical Operator2/2, Logical Operator3/2
  Logical Operator2/1 -> Logical Operator4/2
  In1/1 -> Logical Operator3/1, Logical Operator1/1

== system gates/XOR_basic ==
  In1 : Inport
  In2 : Inport  Port=2
  Logical Operator1 : Logic  IconShape=distinctive  AllPortsSameDT=off  OutDataTypeStr=boolean
  Logical Operator2 : Logic  IconShape=distinctive  AllPortsSameDT=off  OutDataTypeStr=boolean
  Logical Operator3 : Logic  Operator=NOT  IconShape=distinctive  AllPortsSameDT=off  OutDataTypeStr=boolean
  Logical Operator4 : Logic  Operator=OR  IconShape=distinctive  AllPortsSameDT=off  OutDataTypeStr=boolean
  Logical Operator5 : Logic  Operator=NOT  IconShape=distinctive  AllPortsSameDT=off  OutDataTypeStr=boolean
  Out1 : Outport
  wires:
  Logical Operator2/1 -> Logical Operator4/1
  Logical Operator3/1 -> Logical Operator2/1
  Logical Operator1/1 -> Logical Operator4/2
  In1/1 -> Logical Operator3/1, Logical Operator1/1
  Logical Operator4/1 -> Out1/1
  Logical Operator5/1 -> Logical Operator1/2
  In2/1 -> Logical Operator2/2, Logical Operator5/1

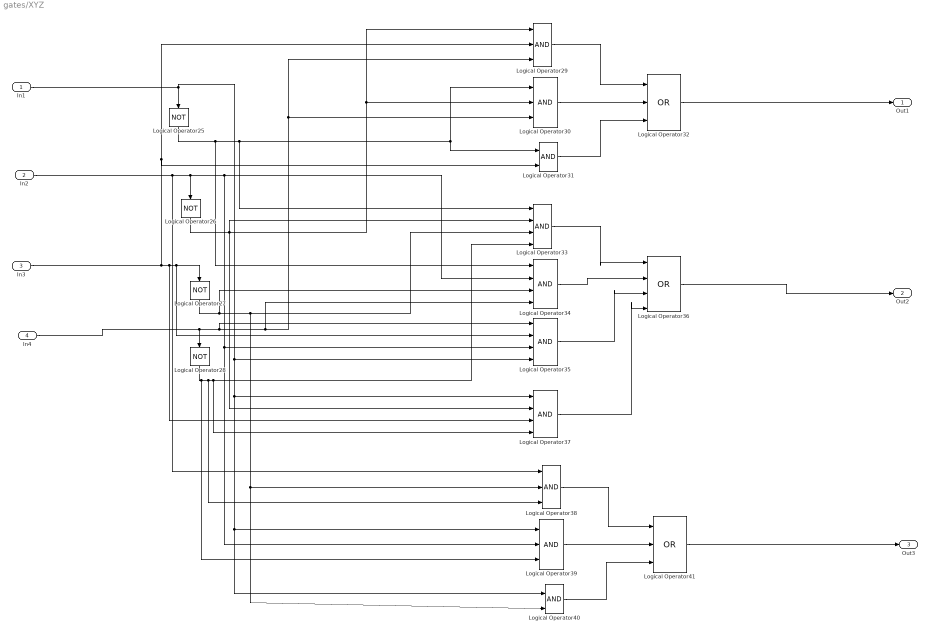
== system gates/XYZ ==
  In1 : Inport
  In2 : Inport  Port=2
  In3 : Inport  Port=3
  In4 : Inport  Port=4
  Logical Operator{25..28} (4 alike) : Logic  Operator=NOT  IconShape=distinctive  AllPortsSameDT=off  OutDataTypeStr=boolean
  Logical Operator{29..30,38..39} (4 alike) : Logic  Inputs=3  IconShape=distinctive  AllPortsSameDT=off  OutDataTypeStr=boolean
  Logical Operator31 : Logic  IconShape=distinctive  AllPortsSameDT=off  OutDataTypeStr=boolean
  Logical Operator32 : Logic  Operator=OR  Inputs=3  IconShape=distinctive  AllPortsSameDT=off  OutDataTypeStr=boolean
  Logical Operator{33..35,37} (4 alike) : Logic  Inputs=4  IconShape=distinctive  AllPortsSameDT=off  OutDataTypeStr=boolean
  Logical Operator36 : Logic  Operator=OR  Inputs=4  IconShape=distinctive  AllPortsSameDT=off  OutDataTypeStr=boolean
  Logical Operator40 : Logic  IconShape=distinctive  AllPortsSameDT=off  OutDataTypeStr=boolean
  Logical Operator41 : Logic  Operator=OR  Inputs=3  IconShape=distinctive  AllPortsSameDT=off  OutDataTypeStr=boolean
  Out1 : Outport
  Out2 : Outport  Port=2
  Out3 : Outport  Port=3
  wires:
  Logical Operator34/1 -> Logical Operator36/2
  In2/1 -> Logical Operator38/1, Logical Operator39/2, Logical Operator35/3, Logical Operator34/2, Logical Operator26/1
  Logical Operator40/1 -> Logical Operator41/3
  In1/1 -> Logical Operator40/1, Logical Operator39/1, Logical Operator37/1, Logical Operator35/4, Logical Operator25/1
  Logical Operator33/1 -> Logical Operator36/1
  In3/1 -> Logical Operator37/3, Logical Operator35/2, Logical Operator27/1, Logical Operator31/2, Logical Operator29/2
  Logical Operator26/1 -> Logical Operator37/2, Logical Operator33/2, Logical Operator30/2, Logical Operator29/1
  Logical Operator41/1 -> Out3/1
  In4/1 -> Logical Operator35/1, Logical Operator34/4, Logical Operator30/3, Logical Operator29/3, Logical Operator28/1
  Logical Operator28/1 -> Logical Operator39/3, Logical Operator38/3, Logical Operator37/4, Logical Operator33/4
  Logical Operator25/1 -> Logical Operator34/1, Logical Operator33/1, Logical Operator30/1, Logical Operator31/1
  Logical Operator30/1 -> Logical Operator32/2
  Logical Operator37/1 -> Logical Operator36/4
  Logical Operator39/1 -> Logical Operator41/2
  Logical Operator27/1 -> Logical Operator40/2, Logical Operator38/2, Logical Operator33/3, Logical Operator34/3
  Logical Operator35/1 -> Logical Operator36/3
  Logical Operator31/1 -> Logical Operator32/3
  Logical Operator29/1 -> Logical Operator32/1
  Logical Operator38/1 -> Logical Operator41/1
  Logical Operator32/1 -> Out1/1
  Logical Operator36/1 -> Out2/1

== system gates/4:1MUX/2:1MUX(Basic)1 ==
  In1 : Inport
  In2 : Inport  Port=2
  In3 : Inport  Port=3
  Logical Operator10 : Logic  IconShape=distinctive  AllPortsSameDT=off  OutDataTypeStr=boolean
  Logical Operator11 : Logic  Operator=NOT  IconShape=distinctive  AllPortsSameDT=off  OutDataTypeStr=boolean
  Logical Operator8 : Logic  IconShape=distinctive  AllPortsSameDT=off  OutDataTypeStr=boolean
  Logical Operator9 : Logic  Operator=OR  IconShape=distinctive  AllPortsSameDT=off  OutDataTypeStr=boolean
  Out1 : Outport
  wires:
  In2/1 -> Logical Operator10/1
  Logical Operator8/1 -> Logical Operator9/1
  Logical Operator9/1 -> Out1/1
  In1/1 -> Logical Operator8/1
  Logical Operator10/1 -> Logical Operator9/2
  Logical Operator11/1 -> Logical Operator8/2
  In3/1 -> Logical Operator10/2, Logical Operator11/1

== system gates/4:1MUX/2:1MUX(Basic)2 ==
  In1 : Inport
  In2 : Inport  Port=2
  In3 : Inport  Port=3
  Logical Operator10 : Logic  IconShape=distinctive  AllPortsSameDT=off  OutDataTypeStr=boolean
  Logical Operator11 : Logic  Operator=NOT  IconShape=distinctive  AllPortsSameDT=off  OutDataTypeStr=boolean
  Logical Operator8 : Logic  IconShape=distinctive  AllPortsSameDT=off  OutDataTypeStr=boolean
  Logical Operator9 : Logic  Operator=OR  IconShape=distinctive  AllPortsSameDT=off  OutDataTypeStr=boolean
  Out1 : Outport
  wires:
  In2/1 -> Logical Operator10/1
  Logical Operator8/1 -> Logical Operator9/1
  Logical Operator9/1 -> Out1/1
  In1/1 -> Logical Operator8/1
  Logical Operator10/1 -> Logical Operator9/2
  Logical Operator11/1 -> Logical Operator8/2
  In3/1 -> Logical Operator10/2, Logical Operator11/1

== system gates/4:1MUX/2:1MUX(Basic)3 ==
  In1 : Inport
  In2 : Inport  Port=2
  In3 : Inport  Port=3
  Logical Operator10 : Logic  IconShape=distinctive  AllPortsSameDT=off  OutDataTypeStr=boolean
  Logical Operator11 : Logic  Operator=NOT  IconShape=distinctive  AllPortsSameDT=off  OutDataTypeStr=boolean
  Logical Operator8 : Logic  IconShape=distinctive  AllPortsSameDT=off  OutDataTypeStr=boolean
  Logical Operator9 : Logic  Operator=OR  IconShape=distinctive  AllPortsSameDT=off  OutDataTypeStr=boolean
  Out1 : Outport
  wires:
  In2/1 -> Logical Operator10/1
  Logical Operator8/1 -> Logical Operator9/1
  Logical Operator9/1 -> Out1/1
  In1/1 -> Logical Operator8/1
  Logical Operator10/1 -> Logical Operator9/2
  Logical Operator11/1 -> Logical Operator8/2
  In3/1 -> Logical Operator10/2, Logical Operator11/1

== system gates/FULLADDER_BASIC/HA_Basic1 ==
  In1 : Inport
  In2 : Inport  Port=2
  Logical Operator2 : Logic  IconShape=distinctive  AllPortsSameDT=off  OutDataTypeStr=boolean
  XOR_basic1 : Subsystem
  Out1 : Outport
  Out2 : Outport  Port=2
  wires:
  XOR_basic1/1(Out1) -> Out1/1
  Logical Operator2/1 -> Out2/1
  In1/1 -> Logical Operator2/1, XOR_basic1/1(In1)
  In2/1 -> Logical Operator2/2, XOR_basic1/2(In2)

== system gates/FULLADDER_BASIC/HA_Basic2 ==
  In1 : Inport
  In2 : Inport  Port=2
  Logical Operator2 : Logic  IconShape=distinctive  AllPortsSameDT=off  OutDataTypeStr=boolean
  XOR_basic1 : Subsystem
  Out1 : Outport
  Out2 : Outport  Port=2
  wires:
  XOR_basic1/1(Out1) -> Out1/1
  Logical Operator2/1 -> Out2/1
  In1/1 -> Logical Operator2/1, XOR_basic1/1(In1)
  In2/1 -> Logical Operator2/2, XOR_basic1/2(In2)

== system gates/HA_Basic/XOR_basic1 ==
  In1 : Inport
  In2 : Inport  Port=2
  Logical Operator1 : Logic  IconShape=distinctive  AllPortsSameDT=off  OutDataTypeStr=boolean
  Logical Operator2 : Logic  IconShape=distinctive  AllPortsSameDT=off  OutDataTypeStr=boolean
  Logical Operator3 : Logic  Operator=NOT  IconShape=distinctive  AllPortsSameDT=off  OutDataTypeStr=boolean
  Logical Operator4 : Logic  Operator=OR  IconShape=distinctive  AllPortsSameDT=off  OutDataTypeStr=boolean
  Logical Operator5 : Logic  Operator=NOT  IconShape=distinctive  AllPortsSameDT=off  OutDataTypeStr=boolean
  Out1 : Outport
  wires:
  Logical Operator2/1 -> Logical Operator4/1
  Logical Operator3/1 -> Logical Operator2/1
  Logical Operator1/1 -> Logical Operator4/2
  In1/1 -> Logical Operator3/1, Logical Operator1/1
  Logical Operator4/1 -> Out1/1
  Logical Operator5/1 -> Logical Operator1/2
  In2/1 -> Logical Operator2/2, Logical Operator5/1

== system gates/HalfAdder_PulseIP/Halfadder_NAND1 ==
  In1 : Inport
  In2 : Inport  Port=2
  Logical Operator1 : Logic  Operator=NAND  IconShape=distinctive  AllPortsSameDT=off  OutDataTypeStr=boolean
  Logical Operator3 : Logic  Operator=NAND  IconShape=distinctive  AllPortsSameDT=off  OutDataTypeStr=boolean
  XOR_Nand1 : Subsystem
  Out1 : Outport
  Out2 : Outport  Port=2
  wires:
  In2/1 -> Logical Operator3/2, XOR_Nand1/2(In2)
  Logical Operator3/1 -> Logical Operator1/2, Logical Operator1/1
  In1/1 -> Logical Operator3/1, XOR_Nand1/1(In1)
  XOR_Nand1/1(Out1) -> Out1/1
  Logical Operator1/1 -> Out2/1

== system gates/Halfadder_NAND/XOR_Nand1 ==
  In1 : Inport
  In2 : Inport  Port=2
  Logical Operator{1..4} (4 alike) : Logic  Operator=NAND  IconShape=distinctive  AllPortsSameDT=off  OutDataTypeStr=boolean
  Out1 : Outport
  wires:
  Logical Operator4/1 -> Out1/1
  Logical Operator1/1 -> Logical Operator4/1
  Logical Operator3/1 -> Logical Operator2/1, Logical Operator1/2
  In2/1 -> Logical Operator2/2, Logical Operator3/2
  Logical Operator2/1 -> Logical Operator4/2
  In1/1 -> Logical Operator3/1, Logical Operator1/1

== system gates/Inrementer/Halfadder_NAND1 ==
  In1 : Inport
  In2 : Inport  Port=2
  Logical Operator1 : Logic  Operator=NAND  IconShape=distinctive  AllPortsSameDT=off  OutDataTypeStr=boolean
  Logical Operator3 : Logic  Operator=NAND  IconShape=distinctive  AllPortsSameDT=off  OutDataTypeStr=boolean
  XOR_Nand1 : Subsystem
  Out1 : Outport
  Out2 : Outport  Port=2
  wires:
  In2/1 -> Logical Operator3/2, XOR_Nand1/2(In2)
  Logical Operator3/1 -> Logical Operator1/2, Logical Operator1/1
  In1/1 -> Logical Operator3/1, XOR_Nand1/1(In1)
  XOR_Nand1/1(Out1) -> Out1/1
  Logical Operator1/1 -> Out2/1

== system gates/Inrementer/Halfadder_NAND2 ==
  In1 : Inport
  In2 : Inport  Port=2
  Logical Operator1 : Logic  Operator=NAND  IconShape=distinctive  AllPortsSameDT=off  OutDataTypeStr=boolean
  Logical Operator3 : Logic  Operator=NAND  IconShape=distinctive  AllPortsSameDT=off  OutDataTypeStr=boolean
  XOR_Nand1 : Subsystem
  Out1 : Outport
  Out2 : Outport  Port=2
  wires:
  In2/1 -> Logical Operator3/2, XOR_Nand1/2(In2)
  Logical Operator3/1 -> Logical Operator1/2, Logical Operator1/1
  In1/1 -> Logical Operator3/1, XOR_Nand1/1(In1)
  XOR_Nand1/1(Out1) -> Out1/1
  Logical Operator1/1 -> Out2/1

== system gates/Inrementer/Halfadder_NAND3 ==
  In1 : Inport
  In2 : Inport  Port=2
  Logical Operator1 : Logic  Operator=NAND  IconShape=distinctive  AllPortsSameDT=off  OutDataTypeStr=boolean
  Logical Operator3 : Logic  Operator=NAND  IconShape=distinctive  AllPortsSameDT=off  OutDataTypeStr=boolean
  XOR_Nand1 : Subsystem
  Out1 : Outport
  Out2 : Outport  Port=2
  wires:
  In2/1 -> Logical Operator3/2, XOR_Nand1/2(In2)
  Logical Operator3/1 -> Logical Operator1/2, Logical Operator1/1
  In1/1 -> Logical Operator3/1, XOR_Nand1/1(In1)
  XOR_Nand1/1(Out1) -> Out1/1
  Logical Operator1/1 -> Out2/1

== system gates/Inrementer/Halfadder_NAND4 ==
  In1 : Inport
  In2 : Inport  Port=2
  Logical Operator1 : Logic  Operator=NAND  IconShape=distinctive  AllPortsSameDT=off  OutDataTypeStr=boolean
  Logical Operator3 : Logic  Operator=NAND  IconShape=distinctive  AllPortsSameDT=off  OutDataTypeStr=boolean
  XOR_Nand1 : Subsystem
  Out1 : Outport
  Out2 : Outport  Port=2
  wires:
  In2/1 -> Logical Operator3/2, XOR_Nand1/2(In2)
  Logical Operator3/1 -> Logical Operator1/2, Logical Operator1/1
  In1/1 -> Logical Operator3/1, XOR_Nand1/1(In1)
  XOR_Nand1/1(Out1) -> Out1/1
  Logical Operator1/1 -> Out2/1

== system gates/PulseIP_XOR/XOR_Nand1 ==
  In1 : Inport
  In2 : Inport  Port=2
  Logical Operator{1..4} (4 alike) : Logic  Operator=NAND  IconShape=distinctive  AllPortsSameDT=off  OutDataTypeStr=boolean
  Out1 : Outport
  wires:
  Logical Operator4/1 -> Out1/1
  Logical Operator1/1 -> Logical Operator4/1
  Logical Operator3/1 -> Logical Operator2/1, Logical Operator1/2
  In2/1 -> Logical Operator2/2, Logical Operator3/2
  Logical Operator2/1 -> Logical Operator4/2
  In1/1 -> Logical Operator3/1, Logical Operator1/1

== system gates/FULLADDER_BASIC/HA_Basic1/XOR_basic1 ==
  In1 : Inport
  In2 : Inport  Port=2
  Logical Operator1 : Logic  IconShape=distinctive  AllPortsSameDT=off  OutDataTypeStr=boolean
  Logical Operator2 : Logic  IconShape=distinctive  AllPortsSameDT=off  OutDataTypeStr=boolean
  Logical Operator3 : Logic  Operator=NOT  IconShape=distinctive  AllPortsSameDT=off  OutDataTypeStr=boolean
  Logical Operator4 : Logic  Operator=OR  IconShape=distinctive  AllPortsSameDT=off  OutDataTypeStr=boolean
  Logical Operator5 : Logic  Operator=NOT  IconShape=distinctive  AllPortsSameDT=off  OutDataTypeStr=boolean
  Out1 : Outport
  wires:
  Logical Operator2/1 -> Logical Operator4/1
  Logical Operator3/1 -> Logical Operator2/1
  Logical Operator1/1 -> Logical Operator4/2
  In1/1 -> Logical Operator3/1, Logical Operator1/1
  Logical Operator4/1 -> Out1/1
  Logical Operator5/1 -> Logical Operator1/2
  In2/1 -> Logical Operator2/2, Logical Operator5/1

== system gates/FULLADDER_BASIC/HA_Basic2/XOR_basic1 ==
  In1 : Inport
  In2 : Inport  Port=2
  Logical Operator1 : Logic  IconShape=distinctive  AllPortsSameDT=off  OutDataTypeStr=boolean
  Logical Operator2 : Logic  IconShape=distinctive  AllPortsSameDT=off  OutDataTypeStr=boolean
  Logical Operator3 : Logic  Operator=NOT  IconShape=distinctive  AllPortsSameDT=off  OutDataTypeStr=boolean
  Logical Operator4 : Logic  Operator=OR  IconShape=distinctive  AllPortsSameDT=off  OutDataTypeStr=boolean
  Logical Operator5 : Logic  Operator=NOT  IconShape=distinctive  AllPortsSameDT=off  OutDataTypeStr=boolean
  Out1 : Outport
  wires:
  Logical Operator2/1 -> Logical Operator4/1
  Logical Operator3/1 -> Logical Operator2/1
  Logical Operator1/1 -> Logical Operator4/2
  In1/1 -> Logical Operator3/1, Logical Operator1/1
  Logical Operator4/1 -> Out1/1
  Logical Operator5/1 -> Logical Operator1/2
  In2/1 -> Logical Operator2/2, Logical Operator5/1

== system gates/HalfAdder_PulseIP/Halfadder_NAND1/XOR_Nand1 ==
  In1 : Inport
  In2 : Inport  Port=2
  Logical Operator{1..4} (4 alike) : Logic  Operator=NAND  IconShape=distinctive  AllPortsSameDT=off  OutDataTypeStr=boolean
  Out1 : Outport
  wires:
  Logical Operator4/1 -> Out1/1
  Logical Operator1/1 -> Logical Operator4/1
  Logical Operator3/1 -> Logical Operator2/1, Logical Operator1/2
  In2/1 -> Logical Operator2/2, Logical Operator3/2
  Logical Operator2/1 -> Logical Operator4/2
  In1/1 -> Logical Operator3/1, Logical Operator1/1

== system gates/Inrementer/Halfadder_NAND1/XOR_Nand1 ==
  In1 : Inport
  In2 : Inport  Port=2
  Logical Operator{1..4} (4 alike) : Logic  Operator=NAND  IconShape=distinctive  AllPortsSameDT=off  OutDataTypeStr=boolean
  Out1 : Outport
  wires:
  Logical Operator4/1 -> Out1/1
  Logical Operator1/1 -> Logical Operator4/1
  Logical Operator3/1 -> Logical Operator2/1, Logical Operator1/2
  In2/1 -> Logical Operator2/2, Logical Operator3/2
  Logical Operator2/1 -> Logical Operator4/2
  In1/1 -> Logical Operator3/1, Logical Operator1/1

== system gates/Inrementer/Halfadder_NAND2/XOR_Nand1 ==
  In1 : Inport
  In2 : Inport  Port=2
  Logical Operator{1..4} (4 alike) : Logic  Operator=NAND  IconShape=distinctive  AllPortsSameDT=off  OutDataTypeStr=boolean
  Out1 : Outport
  wires:
  Logical Operator4/1 -> Out1/1
  Logical Operator1/1 -> Logical Operator4/1
  Logical Operator3/1 -> Logical Operator2/1, Logical Operator1/2
  In2/1 -> Logical Operator2/2, Logical Operator3/2
  Logical Operator2/1 -> Logical Operator4/2
  In1/1 -> Logical Operator3/1, Logical Operator1/1

== system gates/Inrementer/Halfadder_NAND3/XOR_Nand1 ==
  In1 : Inport
  In2 : Inport  Port=2
  Logical Operator{1..4} (4 alike) : Logic  Operator=NAND  IconShape=distinctive  AllPortsSameDT=off  OutDataTypeStr=boolean
  Out1 : Outport
  wires:
  Logical Operator4/1 -> Out1/1
  Logical Operator1/1 -> Logical Operator4/1
  Logical Operator3/1 -> Logical Operator2/1, Logical Operator1/2
  In2/1 -> Logical Operator2/2, Logical Operator3/2
  Logical Operator2/1 -> Logical Operator4/2
  In1/1 -> Logical Operator3/1, Logical Operator1/1

== system gates/Inrementer/Halfadder_NAND4/XOR_Nand1 ==
  In1 : Inport
  In2 : Inport  Port=2
  Logical Operator{1..4} (4 alike) : Logic  Operator=NAND  IconShape=distinctive  AllPortsSameDT=off  OutDataTypeStr=boolean
  Out1 : Outport
  wires:
  Logical Operator4/1 -> Out1/1
  Logical Operator1/1 -> Logical Operator4/1
  Logical Operator3/1 -> Logical Operator2/1, Logical Operator1/2
  In2/1 -> Logical Operator2/2, Logical Operator3/2
  Logical Operator2/1 -> Logical Operator4/2
  In1/1 -> Logical Operator3/1, Logical Operator1/1
